simulink model "block_processing"  (R2023b)
settings: Solver=VariableStepAuto  StartTime=0.0  StopTime=1  RelTol=1e-3
undefined symbols (not defined in the file or in its folder): M, N, none, sz, videoinput
libraries: vipmisc x18, visiontransforms x4, visionstatistics x2, imaqlib x1
settings Model: Creator=luozhongrui  LastModifiedBy=luozhongrui

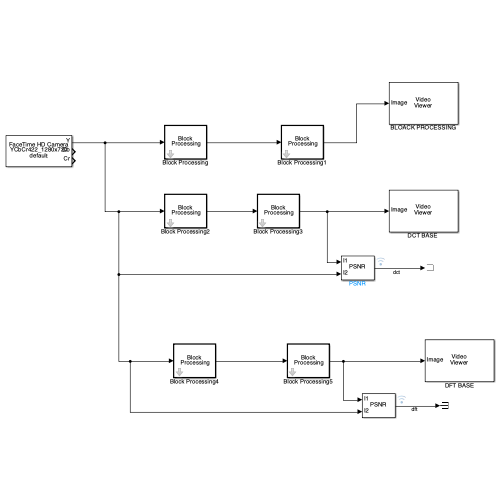
[thumbnail: Simulink's stored preview of the top-level diagram]
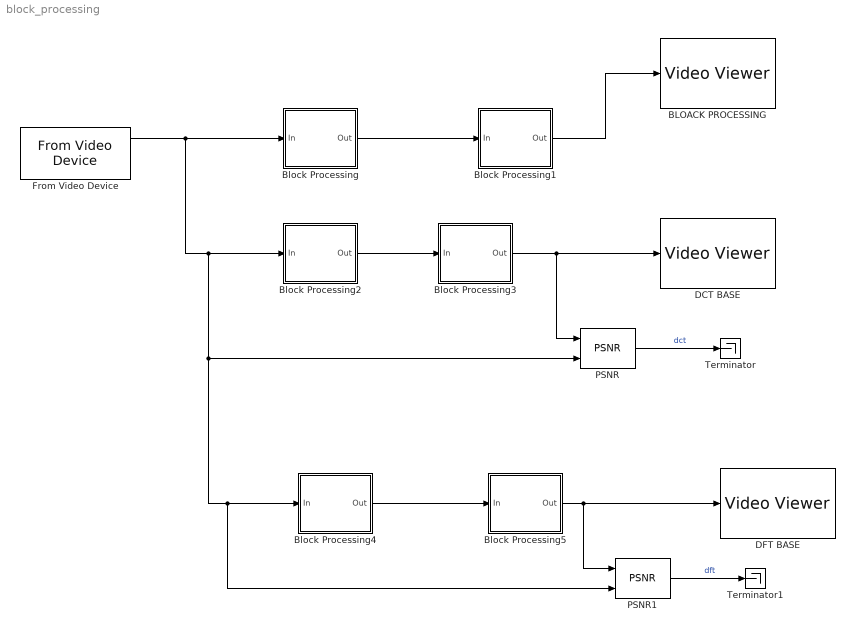
== system block_processing ==
  BLOACK PROCESSING : VideoViewer  FigPos=[661 668 418 304]
  Block Processing : Subsystem  TreatAsAtomicUnit=on  mask(Block Processing){NumI=1, ParamPort=off, NumO=1, Blocksize={[8 8]}, Overlapsize={[0 0]}, Traverse=Row-wise}
      mask prompts: NumI "vision:masks:NumberOfInputs"; ParamPort "vision:masks:AddPortToSupplySubsystemParam"; NumO "vision:masks:NumberOfOutputs"; Blocksize "vision:masks:BlockSize"; Overlapsize "vision:masks:OverlapSize"; Traverse "vision:masks:TraverseOrder"
      mask help: vision:masks:BlockProcessingDescription
      mask init:
      | errmsg = vipblkblockproc(gcbh, NumI, NumO, Blocksize, Overlapsize, Traverse, ParamPort);
      | error(errmsg);
      settings: CopyFcn=set_param(gcb,'LinkStatus','none');
      mask Help: eval('helpview(fullfile(docroot,''toolbox'',''vision'',''vision.map''),''visionblockprocessing'')');
      mask TypeOptions Traverse: vision:masks:Rowwise | vision:masks:Columnwise
      mask DialogControl NumI Prompt: Number of inputs:
      mask DialogControl ParamPort Prompt: Add port to supply subsystem parameters
      mask DialogControl NumO Prompt: Number of outputs:
      mask DialogControl Blocksize Prompt: Block size:
      mask DialogControl Overlapsize Prompt: Overlap size:
      mask DialogControl Traverse Prompt: Traverse order:
      mask DialogControl subsystemGrpBox Prompt: vision:masks:Subsystem
      mask DialogControl subsystemText Prompt: vision:masks:ClickTheOpenSubsystemButton
      mask DialogControl openSubsystem Prompt: vision:masks:OpenSubsystem
      mask DialogControl openSubsystem Callback: Opensubsystem(gcbh)
      mask Display:
      | disp('Block\n Processing');
      | 
      | if ((NumI == 1) && ParamPort)
      |     port_label('input', 1, 'I');
      | end
      | 
      | if (NumI > 1)
      |     for (i = 1:NumI)
      |         port_label('input', i, ['I' int2str(i)]);
      |     end
      | end
      | 
      | if (ParamPort)
      |     port_label('input', NumI+1, 'P');
      | end
  Block Processing1 : Subsystem  TreatAsAtomicUnit=on  mask(Block Processing){NumI=1, ParamPort=off, NumO=1, Blocksize={[8 8]}, Overlapsize={[0 0]}, Traverse=Row-wise}
      mask prompts: NumI "vision:masks:NumberOfInputs"; ParamPort "vision:masks:AddPortToSupplySubsystemParam"; NumO "vision:masks:NumberOfOutputs"; Blocksize "vision:masks:BlockSize"; Overlapsize "vision:masks:OverlapSize"; Traverse "vision:masks:TraverseOrder"
      mask help: vision:masks:BlockProcessingDescription
      mask init:
      | errmsg = vipblkblockproc(gcbh, NumI, NumO, Blocksize, Overlapsize, Traverse, ParamPort);
      | error(errmsg);
      settings: CopyFcn=set_param(gcb,'LinkStatus','none');
      mask Help: eval('helpview(fullfile(docroot,''toolbox'',''vision'',''vision.map''),''visionblockprocessing'')');
      mask TypeOptions Traverse: vision:masks:Rowwise | vision:masks:Columnwise
      mask DialogControl NumI Prompt: Number of inputs:
      mask DialogControl ParamPort Prompt: Add port to supply subsystem parameters
      mask DialogControl NumO Prompt: Number of outputs:
      mask DialogControl Blocksize Prompt: Block size:
      mask DialogControl Overlapsize Prompt: Overlap size:
      mask DialogControl Traverse Prompt: Traverse order:
      mask DialogControl subsystemGrpBox Prompt: vision:masks:Subsystem
      mask DialogControl subsystemText Prompt: vision:masks:ClickTheOpenSubsystemButton
      mask DialogControl openSubsystem Prompt: vision:masks:OpenSubsystem
      mask DialogControl openSubsystem Callback: Opensubsystem(gcbh)
      mask Display:
      | disp('Block\n Processing');
      | 
      | if ((NumI == 1) && ParamPort)
      |     port_label('input', 1, 'I');
      | end
      | 
      | if (NumI > 1)
      |     for (i = 1:NumI)
      |         port_label('input', i, ['I' int2str(i)]);
      |     end
      | end
      | 
      | if (ParamPort)
      |     port_label('input', NumI+1, 'P');
      | end
  Block Processing2 : Subsystem  TreatAsAtomicUnit=on  mask(Block Processing){NumI=1, ParamPort=off, NumO=1, Blocksize={[8 8]}, Overlapsize={[0 0]}, Traverse=Row-wise}
      mask prompts: NumI "vision:masks:NumberOfInputs"; ParamPort "vision:masks:AddPortToSupplySubsystemParam"; NumO "vision:masks:NumberOfOutputs"; Blocksize "vision:masks:BlockSize"; Overlapsize "vision:masks:OverlapSize"; Traverse "vision:masks:TraverseOrder"
      mask help: vision:masks:BlockProcessingDescription
      mask init:
      | errmsg = vipblkblockproc(gcbh, NumI, NumO, Blocksize, Overlapsize, Traverse, ParamPort);
      | error(errmsg);
      settings: CopyFcn=set_param(gcb,'LinkStatus','none');
      mask Help: eval('helpview(fullfile(docroot,''toolbox'',''vision'',''vision.map''),''visionblockprocessing'')');
      mask TypeOptions Traverse: vision:masks:Rowwise | vision:masks:Columnwise
      mask DialogControl NumI Prompt: Number of inputs:
      mask DialogControl ParamPort Prompt: Add port to supply subsystem parameters
      mask DialogControl NumO Prompt: Number of outputs:
      mask DialogControl Blocksize Prompt: Block size:
      mask DialogControl Overlapsize Prompt: Overlap size:
      mask DialogControl Traverse Prompt: Traverse order:
      mask DialogControl subsystemGrpBox Prompt: vision:masks:Subsystem
      mask DialogControl subsystemText Prompt: vision:masks:ClickTheOpenSubsystemButton
      mask DialogControl openSubsystem Prompt: vision:masks:OpenSubsystem
      mask DialogControl openSubsystem Callback: Opensubsystem(gcbh)
      mask Display:
      | disp('Block\n Processing');
      | 
      | if ((NumI == 1) && ParamPort)
      |     port_label('input', 1, 'I');
      | end
      | 
      | if (NumI > 1)
      |     for (i = 1:NumI)
      |         port_label('input', i, ['I' int2str(i)]);
      |     end
      | end
      | 
      | if (ParamPort)
      |     port_label('input', NumI+1, 'P');
      | end
  Block Processing3 : Subsystem  TreatAsAtomicUnit=on  mask(Block Processing){NumI=1, ParamPort=off, NumO=1, Blocksize={[8 8]}, Overlapsize={[0 0]}, Traverse=Row-wise}
      mask prompts: NumI "vision:masks:NumberOfInputs"; ParamPort "vision:masks:AddPortToSupplySubsystemParam"; NumO "vision:masks:NumberOfOutputs"; Blocksize "vision:masks:BlockSize"; Overlapsize "vision:masks:OverlapSize"; Traverse "vision:masks:TraverseOrder"
      mask help: vision:masks:BlockProcessingDescription
      mask init:
      | errmsg = vipblkblockproc(gcbh, NumI, NumO, Blocksize, Overlapsize, Traverse, ParamPort);
      | error(errmsg);
      settings: CopyFcn=set_param(gcb,'LinkStatus','none');
      mask Help: eval('helpview(fullfile(docroot,''toolbox'',''vision'',''vision.map''),''visionblockprocessing'')');
      mask TypeOptions Traverse: vision:masks:Rowwise | vision:masks:Columnwise
      mask DialogControl NumI Prompt: Number of inputs:
      mask DialogControl ParamPort Prompt: Add port to supply subsystem parameters
      mask DialogControl NumO Prompt: Number of outputs:
      mask DialogControl Blocksize Prompt: Block size:
      mask DialogControl Overlapsize Prompt: Overlap size:
      mask DialogControl Traverse Prompt: Traverse order:
      mask DialogControl subsystemGrpBox Prompt: vision:masks:Subsystem
      mask DialogControl subsystemText Prompt: vision:masks:ClickTheOpenSubsystemButton
      mask DialogControl openSubsystem Prompt: vision:masks:OpenSubsystem
      mask DialogControl openSubsystem Callback: Opensubsystem(gcbh)
      mask Display:
      | disp('Block\n Processing');
      | 
      | if ((NumI == 1) && ParamPort)
      |     port_label('input', 1, 'I');
      | end
      | 
      | if (NumI > 1)
      |     for (i = 1:NumI)
      |         port_label('input', i, ['I' int2str(i)]);
      |     end
      | end
      | 
      | if (ParamPort)
      |     port_label('input', NumI+1, 'P');
      | end
  Block Processing4 : Subsystem  TreatAsAtomicUnit=on  mask(Block Processing){NumI=1, ParamPort=off, NumO=1, Blocksize={[8 8]}, Overlapsize={[0 0]}, Traverse=Row-wise}
      mask prompts: NumI "vision:masks:NumberOfInputs"; ParamPort "vision:masks:AddPortToSupplySubsystemParam"; NumO "vision:masks:NumberOfOutputs"; Blocksize "vision:masks:BlockSize"; Overlapsize "vision:masks:OverlapSize"; Traverse "vision:masks:TraverseOrder"
      mask help: vision:masks:BlockProcessingDescription
      mask init:
      | errmsg = vipblkblockproc(gcbh, NumI, NumO, Blocksize, Overlapsize, Traverse, ParamPort);
      | error(errmsg);
      settings: CopyFcn=set_param(gcb,'LinkStatus','none');
      mask Help: eval('helpview(fullfile(docroot,''toolbox'',''vision'',''vision.map''),''visionblockprocessing'')');
      mask TypeOptions Traverse: vision:masks:Rowwise | vision:masks:Columnwise
      mask DialogControl NumI Prompt: Number of inputs:
      mask DialogControl ParamPort Prompt: Add port to supply subsystem parameters
      mask DialogControl NumO Prompt: Number of outputs:
      mask DialogControl Blocksize Prompt: Block size:
      mask DialogControl Overlapsize Prompt: Overlap size:
      mask DialogControl Traverse Prompt: Traverse order:
      mask DialogControl subsystemGrpBox Prompt: vision:masks:Subsystem
      mask DialogControl subsystemText Prompt: vision:masks:ClickTheOpenSubsystemButton
      mask DialogControl openSubsystem Prompt: vision:masks:OpenSubsystem
      mask DialogControl openSubsystem Callback: Opensubsystem(gcbh)
      mask Display:
      | disp('Block\n Processing');
      | 
      | if ((NumI == 1) && ParamPort)
      |     port_label('input', 1, 'I');
      | end
      | 
      | if (NumI > 1)
      |     for (i = 1:NumI)
      |         port_label('input', i, ['I' int2str(i)]);
      |     end
      | end
      | 
      | if (ParamPort)
      |     port_label('input', NumI+1, 'P');
      | end
  Block Processing5 : Subsystem  TreatAsAtomicUnit=on  mask(Block Processing){NumI=1, ParamPort=off, NumO=1, Blocksize={[8 8]}, Overlapsize={[0 0]}, Traverse=Row-wise}
      mask prompts: NumI "vision:masks:NumberOfInputs"; ParamPort "vision:masks:AddPortToSupplySubsystemParam"; NumO "vision:masks:NumberOfOutputs"; Blocksize "vision:masks:BlockSize"; Overlapsize "vision:masks:OverlapSize"; Traverse "vision:masks:TraverseOrder"
      mask help: vision:masks:BlockProcessingDescription
      mask init:
      | errmsg = vipblkblockproc(gcbh, NumI, NumO, Blocksize, Overlapsize, Traverse, ParamPort);
      | error(errmsg);
      settings: CopyFcn=set_param(gcb,'LinkStatus','none');
      mask Help: eval('helpview(fullfile(docroot,''toolbox'',''vision'',''vision.map''),''visionblockprocessing'')');
      mask TypeOptions Traverse: vision:masks:Rowwise | vision:masks:Columnwise
      mask DialogControl NumI Prompt: Number of inputs:
      mask DialogControl ParamPort Prompt: Add port to supply subsystem parameters
      mask DialogControl NumO Prompt: Number of outputs:
      mask DialogControl Blocksize Prompt: Block size:
      mask DialogControl Overlapsize Prompt: Overlap size:
      mask DialogControl Traverse Prompt: Traverse order:
      mask DialogControl subsystemGrpBox Prompt: vision:masks:Subsystem
      mask DialogControl subsystemText Prompt: vision:masks:ClickTheOpenSubsystemButton
      mask DialogControl openSubsystem Prompt: vision:masks:OpenSubsystem
      mask DialogControl openSubsystem Callback: Opensubsystem(gcbh)
      mask Display:
      | disp('Block\n Processing');
      | 
      | if ((NumI == 1) && ParamPort)
      |     port_label('input', 1, 'I');
      | end
      | 
      | if (NumI > 1)
      |     for (i = 1:NumI)
      |         port_label('input', i, ['I' int2str(i)]);
      |     end
      | end
      | 
      | if (ParamPort)
      |     port_label('input', NumI+1, 'P');
      | end
  "DCT BASE " : VideoViewer  FigPos=[213 604 418 304]
  DFT BASE : VideoViewer  FigPos=[597 705 418 304]
  From Video Device : imaqlib/From Video Device  DeviceMenu=macvideo 1 (FaceTime HD Camera)  Device=macvideo 1 (FaceTime HD Camera)  ObjConstructor=videoinput('macvideo', 1)  VideoFormatMenu=YCbCr422_1280x720  VideoFormat=YCbCr422_1280x720  VideoSource=default  ROIPosition=[0 0 720 1280]  EnableHWTrigger=off  TriggerConfiguration=none/none  SampleTime=1/30  OutputPortsMode=Separate color signals  DataType=single  CanDoHWTrigger=no  ReturnedColorSpace=YCbCr  BlockHandle=4.0002  ROIWidth=1280  ROIHeight=720  ROIColumn=0  ROIRow=0  EngXMLPath=/Applications/MATLAB_R2023b.app/toolbox/imaq/imaq/private  DevXMLPath=/Users/luozhongrui/Documents/MATLAB/SupportPackages/R2023b/toolbox/imaq/supportpackages/genericvideo/adaptor/maca64  EngLibPath=/Applications/MATLAB_R2023b.app/toolbox/imaq/imaqblks/imaqmex/maca64  ColorSpace=YCbCr  BayerSensorAlignment=grbg  ImaqMode=off
  PSNR : visionstatistics/PSNR
  PSNR1 : visionstatistics/PSNR
  Terminator : Terminator
  Terminator1 : Terminator
  wires:
  From Video Device/1 -> PSNR1/2, Block Processing4/1(In), PSNR/2, Block Processing2/1(In), Block Processing/1(In)
  Block Processing1/1(Out) -> BLOACK PROCESSING/1
  Block Processing/1(Out) -> Block Processing1/1(In)
  Block Processing2/1(Out) -> Block Processing3/1(In)
  Block Processing3/1(Out) -> PSNR/1, "DCT BASE "/1
  PSNR/1 -> Terminator/1  "dct"
  Block Processing4/1(Out) -> Block Processing5/1(In)
  Block Processing5/1(Out) -> PSNR1/1, DFT BASE/1
  PSNR1/1 -> Terminator1/1  "dft"

== system block_processing/Block Processing ==
  In : Inport
  Block iterator : Subsystem
      settings: CopyFcn=set_param(gcb,'ReferenceBlock','');
  Iteration count : vipmisc/Iteration count  NumI=NumI  blksize=Blocksize  ovlpsize=Overlapsize
  Out : Outport  VectorParamsAs1DForOutWhenUnconnected=off
  wires:
  Iteration count/1 -> Block iterator/1(iter)
  In/1 -> Iteration count/1, Block iterator/2(In1)
  Block iterator/1(Out) -> Out/1

== system block_processing/Block Processing1 ==
  In : Inport
  Block iterator : Subsystem
      settings: CopyFcn=set_param(gcb,'ReferenceBlock','');
  Iteration count : vipmisc/Iteration count  NumI=NumI  blksize=Blocksize  ovlpsize=Overlapsize
  Out : Outport  VectorParamsAs1DForOutWhenUnconnected=off
  wires:
  Iteration count/1 -> Block iterator/1(iter)
  In/1 -> Iteration count/1, Block iterator/2(In1)
  Block iterator/1(Out) -> Out/1

== system block_processing/Block Processing2 ==
  In : Inport
  Block iterator : Subsystem
      settings: CopyFcn=set_param(gcb,'ReferenceBlock','');
  Iteration count : vipmisc/Iteration count  NumI=NumI  blksize=Blocksize  ovlpsize=Overlapsize
  Out : Outport  VectorParamsAs1DForOutWhenUnconnected=off
  wires:
  Iteration count/1 -> Block iterator/1(iter)
  In/1 -> Iteration count/1, Block iterator/2(In1)
  Block iterator/1(Out) -> Out/1

== system block_processing/Block Processing3 ==
  In : Inport
  Block iterator : Subsystem
      settings: CopyFcn=set_param(gcb,'ReferenceBlock','');
  Iteration count : vipmisc/Iteration count  NumI=NumI  blksize=Blocksize  ovlpsize=Overlapsize
  Out : Outport  VectorParamsAs1DForOutWhenUnconnected=off
  wires:
  Iteration count/1 -> Block iterator/1(iter)
  In/1 -> Iteration count/1, Block iterator/2(In1)
  Block iterator/1(Out) -> Out/1

== system block_processing/Block Processing4 ==
  In : Inport
  Block iterator : Subsystem
      settings: CopyFcn=set_param(gcb,'ReferenceBlock','');
  Iteration count : vipmisc/Iteration count  NumI=NumI  blksize=Blocksize  ovlpsize=Overlapsize
  Out : Outport  VectorParamsAs1DForOutWhenUnconnected=off
  wires:
  Iteration count/1 -> Block iterator/1(iter)
  In/1 -> Iteration count/1, Block iterator/2(In1)
  Block iterator/1(Out) -> Out/1

== system block_processing/Block Processing5 ==
  In : Inport
  Block iterator : Subsystem
      settings: CopyFcn=set_param(gcb,'ReferenceBlock','');
  Iteration count : vipmisc/Iteration count  NumI=NumI  blksize=Blocksize  ovlpsize=Overlapsize
  Out : Outport  VectorParamsAs1DForOutWhenUnconnected=off
  wires:
  Iteration count/1 -> Block iterator/1(iter)
  In/1 -> Iteration count/1, Block iterator/2(In1)
  Block iterator/1(Out) -> Out/1

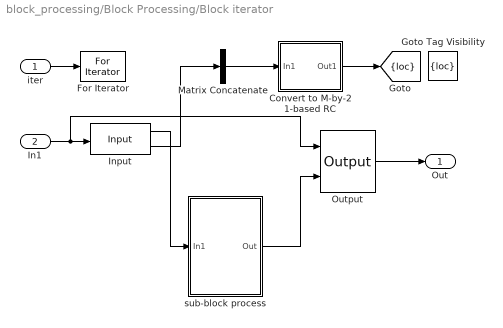
== system block_processing/Block Processing/Block iterator ==
  iter : Inport
  In1 : Inport  Port=2
  Convert to M-by-2 1-based RC : Subsystem
  For Iterator : ForIterator  IterationSource=external  IterationLimit=(sz(1)/M)*(sz(2)/N)  ShowIterationPort=off  IndexMode=Zero-based  IterationVariableDataType=double
  Goto Tag Visibility : GotoTagVisibility  GotoTag=loc
  Input : vipmisc/Input  Blocksize=Blocksize{1}  Overlapsize=Overlapsize{1}  tverse=Row-wise
  Matrix Concatenate : Concatenate  NumInputs=1  Mode=Multidimensional array  ConcatenateDimension=2
  Output : vipmisc/Output  Blocksize=Blocksize{1}  Overlapsize=Overlapsize{1}  tverse=Row-wise
  sub-block process : Subsystem
  Out : Outport  VectorParamsAs1DForOutWhenUnconnected=off
  tag scope: loc=scoped
  wires:
  Convert to M-by-2 1-based RC/1(Out1) -> [loc]
  Matrix Concatenate/1 -> Convert to M-by-2 1-based RC/1(In1)
  Input/2 -> Matrix Concatenate/1
  Input/1 -> sub-block process/1(In1)
  iter/1 -> For Iterator/1
  In1/1 -> Input/1, Output/1
  Output/1 -> Out/1
  sub-block process/1(Out) -> Output/2

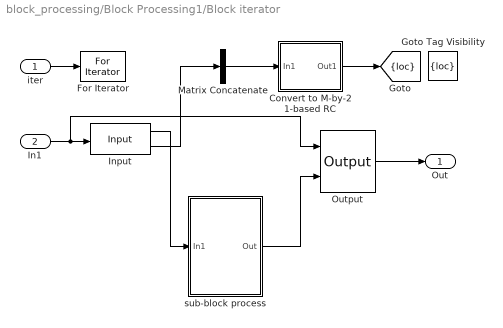
== system block_processing/Block Processing1/Block iterator ==
  iter : Inport
  In1 : Inport  Port=2
  Convert to M-by-2 1-based RC : Subsystem
  For Iterator : ForIterator  IterationSource=external  IterationLimit=(sz(1)/M)*(sz(2)/N)  ShowIterationPort=off  IndexMode=Zero-based  IterationVariableDataType=double
  Goto Tag Visibility : GotoTagVisibility  GotoTag=loc
  Input : vipmisc/Input  Blocksize=Blocksize{1}  Overlapsize=Overlapsize{1}  tverse=Row-wise
  Matrix Concatenate : Concatenate  NumInputs=1  Mode=Multidimensional array  ConcatenateDimension=2
  Output : vipmisc/Output  Blocksize=Blocksize{1}  Overlapsize=Overlapsize{1}  tverse=Row-wise
  sub-block process : Subsystem
  Out : Outport  VectorParamsAs1DForOutWhenUnconnected=off
  tag scope: loc=scoped
  wires:
  Convert to M-by-2 1-based RC/1(Out1) -> [loc]
  Matrix Concatenate/1 -> Convert to M-by-2 1-based RC/1(In1)
  Input/2 -> Matrix Concatenate/1
  Input/1 -> sub-block process/1(In1)
  iter/1 -> For Iterator/1
  In1/1 -> Input/1, Output/1
  Output/1 -> Out/1
  sub-block process/1(Out) -> Output/2

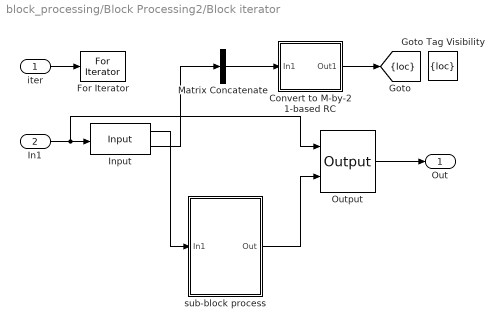
== system block_processing/Block Processing2/Block iterator ==
  iter : Inport
  In1 : Inport  Port=2
  Convert to M-by-2 1-based RC : Subsystem
  For Iterator : ForIterator  IterationSource=external  IterationLimit=(sz(1)/M)*(sz(2)/N)  ShowIterationPort=off  IndexMode=Zero-based  IterationVariableDataType=double
  Goto Tag Visibility : GotoTagVisibility  GotoTag=loc
  Input : vipmisc/Input  Blocksize=Blocksize{1}  Overlapsize=Overlapsize{1}  tverse=Row-wise
  Matrix Concatenate : Concatenate  NumInputs=1  Mode=Multidimensional array  ConcatenateDimension=2
  Output : vipmisc/Output  Blocksize=Blocksize{1}  Overlapsize=Overlapsize{1}  tverse=Row-wise
  sub-block process : Subsystem
  Out : Outport  VectorParamsAs1DForOutWhenUnconnected=off
  tag scope: loc=scoped
  wires:
  Convert to M-by-2 1-based RC/1(Out1) -> [loc]
  Matrix Concatenate/1 -> Convert to M-by-2 1-based RC/1(In1)
  Input/2 -> Matrix Concatenate/1
  Input/1 -> sub-block process/1(In1)
  iter/1 -> For Iterator/1
  In1/1 -> Input/1, Output/1
  Output/1 -> Out/1
  sub-block process/1(Out) -> Output/2

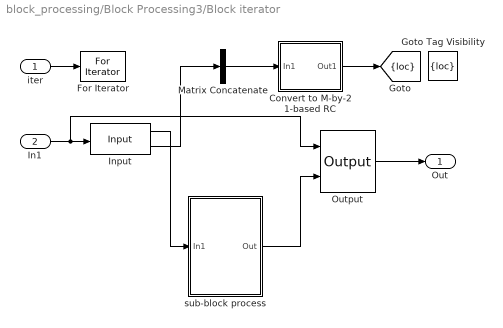
== system block_processing/Block Processing3/Block iterator ==
  iter : Inport
  In1 : Inport  Port=2
  Convert to M-by-2 1-based RC : Subsystem
  For Iterator : ForIterator  IterationSource=external  IterationLimit=(sz(1)/M)*(sz(2)/N)  ShowIterationPort=off  IndexMode=Zero-based  IterationVariableDataType=double
  Goto Tag Visibility : GotoTagVisibility  GotoTag=loc
  Input : vipmisc/Input  Blocksize=Blocksize{1}  Overlapsize=Overlapsize{1}  tverse=Row-wise
  Matrix Concatenate : Concatenate  NumInputs=1  Mode=Multidimensional array  ConcatenateDimension=2
  Output : vipmisc/Output  Blocksize=Blocksize{1}  Overlapsize=Overlapsize{1}  tverse=Row-wise
  sub-block process : Subsystem
  Out : Outport  VectorParamsAs1DForOutWhenUnconnected=off
  tag scope: loc=scoped
  wires:
  Convert to M-by-2 1-based RC/1(Out1) -> [loc]
  Matrix Concatenate/1 -> Convert to M-by-2 1-based RC/1(In1)
  Input/2 -> Matrix Concatenate/1
  Input/1 -> sub-block process/1(In1)
  iter/1 -> For Iterator/1
  In1/1 -> Input/1, Output/1
  Output/1 -> Out/1
  sub-block process/1(Out) -> Output/2

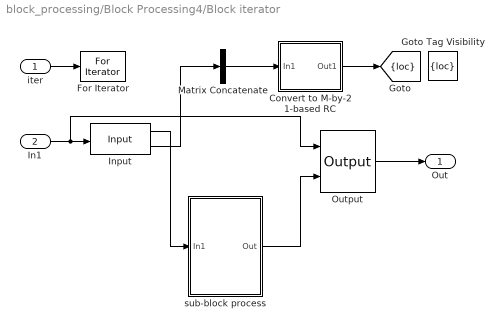
== system block_processing/Block Processing4/Block iterator ==
  iter : Inport
  In1 : Inport  Port=2
  Convert to M-by-2 1-based RC : Subsystem
  For Iterator : ForIterator  IterationSource=external  IterationLimit=(sz(1)/M)*(sz(2)/N)  ShowIterationPort=off  IndexMode=Zero-based  IterationVariableDataType=double
  Goto Tag Visibility : GotoTagVisibility  GotoTag=loc
  Input : vipmisc/Input  Blocksize=Blocksize{1}  Overlapsize=Overlapsize{1}  tverse=Row-wise
  Matrix Concatenate : Concatenate  NumInputs=1  Mode=Multidimensional array  ConcatenateDimension=2
  Output : vipmisc/Output  Blocksize=Blocksize{1}  Overlapsize=Overlapsize{1}  tverse=Row-wise
  sub-block process : Subsystem
  Out : Outport  VectorParamsAs1DForOutWhenUnconnected=off
  tag scope: loc=scoped
  wires:
  Convert to M-by-2 1-based RC/1(Out1) -> [loc]
  Matrix Concatenate/1 -> Convert to M-by-2 1-based RC/1(In1)
  Input/2 -> Matrix Concatenate/1
  Input/1 -> sub-block process/1(In1)
  iter/1 -> For Iterator/1
  In1/1 -> Input/1, Output/1
  Output/1 -> Out/1
  sub-block process/1(Out) -> Output/2

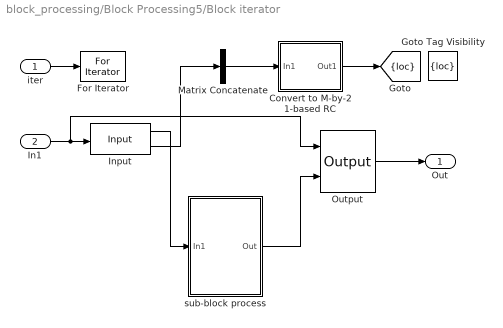
== system block_processing/Block Processing5/Block iterator ==
  iter : Inport
  In1 : Inport  Port=2
  Convert to M-by-2 1-based RC : Subsystem
  For Iterator : ForIterator  IterationSource=external  IterationLimit=(sz(1)/M)*(sz(2)/N)  ShowIterationPort=off  IndexMode=Zero-based  IterationVariableDataType=double
  Goto Tag Visibility : GotoTagVisibility  GotoTag=loc
  Input : vipmisc/Input  Blocksize=Blocksize{1}  Overlapsize=Overlapsize{1}  tverse=Row-wise
  Matrix Concatenate : Concatenate  NumInputs=1  Mode=Multidimensional array  ConcatenateDimension=2
  Output : vipmisc/Output  Blocksize=Blocksize{1}  Overlapsize=Overlapsize{1}  tverse=Row-wise
  sub-block process : Subsystem
  Out : Outport  VectorParamsAs1DForOutWhenUnconnected=off
  tag scope: loc=scoped
  wires:
  Convert to M-by-2 1-based RC/1(Out1) -> [loc]
  Matrix Concatenate/1 -> Convert to M-by-2 1-based RC/1(In1)
  Input/2 -> Matrix Concatenate/1
  Input/1 -> sub-block process/1(In1)
  iter/1 -> For Iterator/1
  In1/1 -> Input/1, Output/1
  Output/1 -> Out/1
  sub-block process/1(Out) -> Output/2

== system block_processing/Block Processing/Block iterator/Convert to M-by-2 1-based RC ==
  In1 : Inport
  Bias : Bias  Bias=1  SaturateOnIntegerOverflow=off
  Permute Dimensions : PermuteDimensions
  Out1 : Outport  VectorParamsAs1DForOutWhenUnconnected=off
  wires:
  In1/1 -> Permute Dimensions/1
  Bias/1 -> Out1/1
  Permute Dimensions/1 -> Bias/1

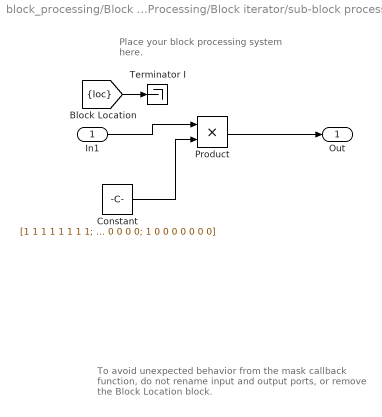
== system block_processing/Block Processing/Block iterator/sub-block process ==
  note: To avoid unexpected behavior from the mask
      | callback function, do not rename input and output ports,
      | or remove the Block Location block.
  note: Place your block
      | processing system here.
  In1 : Inport
  Constant : Constant  Value=[1 1 1 1 1 1 1 1; 1 1 1 1 1 1 1 0; 1 1 1 1 1 1 0 0; 1 1 1 1 1 0 0 0; 1 1 1 1 0 0 0 0; 1 1 1 0 0 0 0 0; 1 1 0 0 0 0 0 0; 1 0 0 0 0 0 0 0]
  Product : Product
  Terminator I : Terminator
  Out : Outport  VectorParamsAs1DForOutWhenUnconnected=off
  wires:
  [loc] -> Terminator I/1
  Product/1 -> Out/1
  In1/1 -> Product/1
  Constant/1 -> Product/2

== system block_processing/Block Processing1/Block iterator/Convert to M-by-2 1-based RC ==
  In1 : Inport
  Bias : Bias  Bias=1  SaturateOnIntegerOverflow=off
  Permute Dimensions : PermuteDimensions
  Out1 : Outport  VectorParamsAs1DForOutWhenUnconnected=off
  wires:
  In1/1 -> Permute Dimensions/1
  Bias/1 -> Out1/1
  Permute Dimensions/1 -> Bias/1

== system block_processing/Block Processing1/Block iterator/sub-block process ==
  note: To avoid unexpected behavior from the mask
      | callback function, do not rename input and output ports,
      | or remove the Block Location block.
  note: Place your block
      | processing system here.
  In1 : Inport
  Terminator I : Terminator
  Out : Outport  VectorParamsAs1DForOutWhenUnconnected=off
  wires:
  [loc] -> Terminator I/1
  In1/1 -> Out/1

== system block_processing/Block Processing2/Block iterator/Convert to M-by-2 1-based RC ==
  In1 : Inport
  Bias : Bias  Bias=1  SaturateOnIntegerOverflow=off
  Permute Dimensions : PermuteDimensions
  Out1 : Outport  VectorParamsAs1DForOutWhenUnconnected=off
  wires:
  In1/1 -> Permute Dimensions/1
  Bias/1 -> Out1/1
  Permute Dimensions/1 -> Bias/1

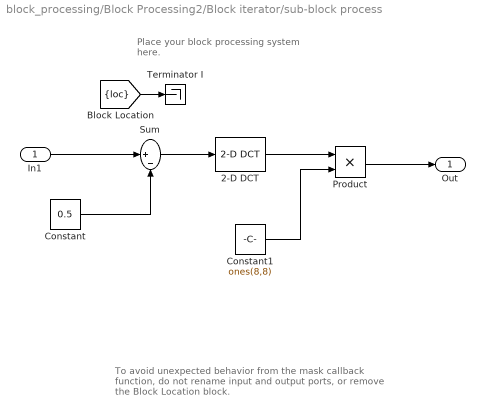
== system block_processing/Block Processing2/Block iterator/sub-block process ==
  note: To avoid unexpected behavior from the mask
      | callback function, do not rename input and output ports,
      | or remove the Block Location block.
  note: Place your block
      | processing system here.
  In1 : Inport
  2-D DCT : visiontransforms/2-D DCT  CompMethod=Table lookup  Dimension=0  TableOpt=Speed  BitRevOrder=off  SkipNorm=off  firstCoeffLastDataTypeStr=Inherit: Same word length as input  roundingMode=Floor  overflowMode=off  firstCoeffDataTypeStr=Inherit: Same word length as input  outputMin=[]  outputMax=[]
  Constant : Constant  Value=0.5
  Constant1 : Constant  Value=ones(8,8)  VectorParams1D=off
  Product : Product
  Sum : Sum  Inputs=|+-
  Terminator I : Terminator
  Out : Outport  VectorParamsAs1DForOutWhenUnconnected=off
  wires:
  [loc] -> Terminator I/1
  Constant/1 -> Sum/2
  In1/1 -> Sum/1
  Sum/1 -> 2-D DCT/1
  2-D DCT/1 -> Product/1
  Constant1/1 -> Product/2
  Product/1 -> Out/1

== system block_processing/Block Processing3/Block iterator/Convert to M-by-2 1-based RC ==
  In1 : Inport
  Bias : Bias  Bias=1  SaturateOnIntegerOverflow=off
  Permute Dimensions : PermuteDimensions
  Out1 : Outport  VectorParamsAs1DForOutWhenUnconnected=off
  wires:
  In1/1 -> Permute Dimensions/1
  Bias/1 -> Out1/1
  Permute Dimensions/1 -> Bias/1

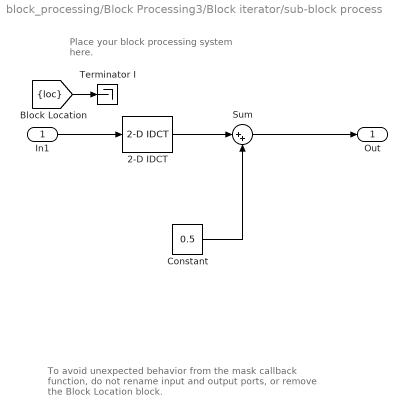
== system block_processing/Block Processing3/Block iterator/sub-block process ==
  note: To avoid unexpected behavior from the mask
      | callback function, do not rename input and output ports,
      | or remove the Block Location block.
  note: Place your block
      | processing system here.
  In1 : Inport
  2-D IDCT : visiontransforms/2-D IDCT  CompMethod=Table lookup  Dimension=0  TableOpt=Speed  BitRevOrder=off  SkipNorm=off  firstCoeffLastDataTypeStr=Inherit: Same word length as input  roundingMode=Floor  overflowMode=off  firstCoeffDataTypeStr=Inherit: Same word length as input  outputMin=[]  outputMax=[]
  Constant : Constant  Value=0.5
  Sum : Sum  Inputs=|++  OutDataTypeStr=single
  Terminator I : Terminator
  Out : Outport  VectorParamsAs1DForOutWhenUnconnected=off
  wires:
  [loc] -> Terminator I/1
  In1/1 -> 2-D IDCT/1
  2-D IDCT/1 -> Sum/1
  Constant/1 -> Sum/2
  Sum/1 -> Out/1

== system block_processing/Block Processing4/Block iterator/Convert to M-by-2 1-based RC ==
  In1 : Inport
  Bias : Bias  Bias=1  SaturateOnIntegerOverflow=off
  Permute Dimensions : PermuteDimensions
  Out1 : Outport  VectorParamsAs1DForOutWhenUnconnected=off
  wires:
  In1/1 -> Permute Dimensions/1
  Bias/1 -> Out1/1
  Permute Dimensions/1 -> Bias/1

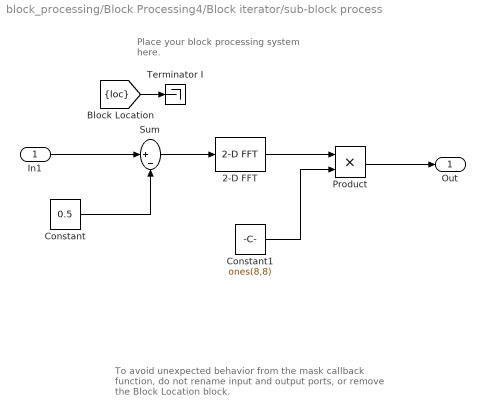
== system block_processing/Block Processing4/Block iterator/sub-block process ==
  note: To avoid unexpected behavior from the mask
      | callback function, do not rename input and output ports,
      | or remove the Block Location block.
  note: Place your block
      | processing system here.
  In1 : Inport
  2-D FFT : visiontransforms/2-D FFT  TableOpt=NEW  TableOptActive=Speed  FFTImplementation=Auto  BitRevOrder=off  SkipNorm=off  firstCoeffLastDataTypeStr=Inherit: Same word length as input  roundingMode=Floor  overflowMode=off  firstCoeffDataTypeStr=Inherit: Same word length as input  outputMin=[]  outputMax=[]
  Constant : Constant  Value=0.5
  Constant1 : Constant  Value=ones(8,8)  VectorParams1D=off
  Product : Product
  Sum : Sum  Inputs=|+-
  Terminator I : Terminator
  Out : Outport  VectorParamsAs1DForOutWhenUnconnected=off
  wires:
  [loc] -> Terminator I/1
  Constant/1 -> Sum/2
  In1/1 -> Sum/1
  Sum/1 -> 2-D FFT/1
  2-D FFT/1 -> Product/1
  Constant1/1 -> Product/2
  Product/1 -> Out/1

== system block_processing/Block Processing5/Block iterator/Convert to M-by-2 1-based RC ==
  In1 : Inport
  Bias : Bias  Bias=1  SaturateOnIntegerOverflow=off
  Permute Dimensions : PermuteDimensions
  Out1 : Outport  VectorParamsAs1DForOutWhenUnconnected=off
  wires:
  In1/1 -> Permute Dimensions/1
  Bias/1 -> Out1/1
  Permute Dimensions/1 -> Bias/1

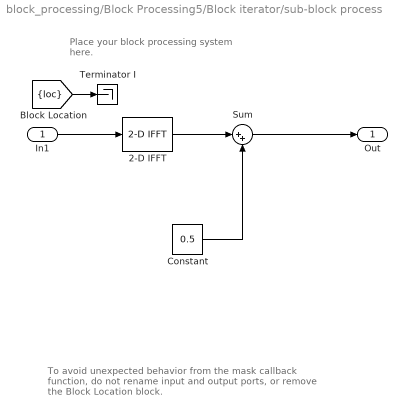
== system block_processing/Block Processing5/Block iterator/sub-block process ==
  note: To avoid unexpected behavior from the mask
      | callback function, do not rename input and output ports,
      | or remove the Block Location block.
  note: Place your block
      | processing system here.
  In1 : Inport
  2-D IFFT : visiontransforms/2-D IFFT  TableOpt=NEW  TableOptActive=Speed  FFTImplementation=Auto  BitRevOrder=off  cs_in=on  divideOutput=on  SkipNorm=on  firstCoeffLastDataTypeStr=Inherit: Same word length as input  roundingMode=Floor  overflowMode=off  firstCoeffDataTypeStr=Inherit: Same word length as input  outputMin=[]  outputMax=[]
  Constant : Constant  Value=0.5
  Sum : Sum  Inputs=|++  OutDataTypeStr=single
  Terminator I : Terminator
  Out : Outport  VectorParamsAs1DForOutWhenUnconnected=off
  wires:
  [loc] -> Terminator I/1
  In1/1 -> 2-D IFFT/1
  2-D IFFT/1 -> Sum/1
  Constant/1 -> Sum/2
  Sum/1 -> Out/1
